simulink model "spe_engine_throttle1"  (R2020a)
settings: Solver=ode45  StartTime=0  StopTime=0.5  FixedStep=.001  RelTol=1e-3  EnableMultiTasking=on
PreLoadFcn:
  | load spe_engine_throttle1.mat
model workspace (MAT data in the model file):
  spe_engine_throttle1_spesession : sldodialogs.data.SessionData (value not decoded)
undefined symbols (not defined in the file): angle_init, angle_open, c, input_delay, J, k, Kt
settings Model: Creator=The MathWorks, Inc.  LastModifiedBy=GreHiDel
settings SolverCC: ZeroCrossAlgorithm=Classic  InsertRTBMode=Auto
settings DataIOCC: ExternalInput=[time1,input1]  LoadExternalInput=on  SaveFormat=Array  SaveOutput=off  SaveTime=off  ReturnWorkspaceOutputs=off
settings OptimizationCC: BooleanDataType=off  ExpressionDepthLimit=2147483647  InitFltsAndDblsToZero=on  LifeSpan=inf  BufferReusableBoundary=off
settings DebuggingCC: SaveWithParameterizedLinksMsg=none  UnderspecifiedInitializationDetection=Classic  MergeDetectMultiDrivingBlocksExec=none  SignalResolutionControl=TryResolveAllWithWarning  MultiTaskDSMMsg=warning  MultiTaskCondExecSysMsg=none  FcnCallInpInsideContextMsg=warning  BusObjectLabelMismatch=none  StateNameClashWarn=warning  SFUnexpectedBacktrackingDiag=warning  SFNoUnconditionalDefaultTransitionDiag=warning  SFExecutionAtInitializationDiag=none  ArithmeticOperatorsInVariantConditions=warning
settings HardwareCC: ProdBitPerPointer=32  ProdBitPerSizeT=32  ProdBitPerPtrDiffT=32  ProdLargestAtomicFloat=None  ProdIntDivRoundTo=Undefined  ProdEndianess=Unspecified  ProdWordSize=32  ProdHWDeviceType=32-bit Generic  TargetUnknown=on
settings ModelReferenceCC: PropagateSignalLabelsOutOfModel=off
settings CodeAppCC: StateflowObjectComments=on
settings GRTTargetCC: TargetFcnLib=ansi_tfl_tmw.mat  TargetLangStandard=C89/C90 (ANSI)  CombineOutputUpdateFcns=off  GRTInterface=on
settings ConfigComp: CovMetricSettings=dw  CovHtmlReporting=on  CovSaveCumulativeToWorkspaceVar=on  CovSaveSingleToWorkspaceVar=on

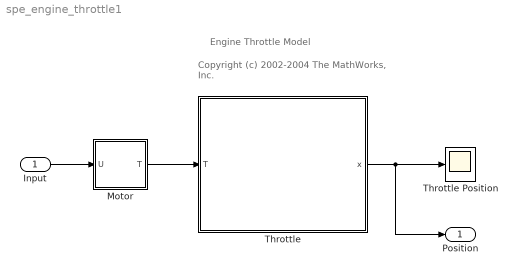
== system spe_engine_throttle1 ==
  note: Engine Throttle Model
  note: Copyright (c) 2002-2004 The MathWorks, Inc.
  Input : Inport
  Motor : Subsystem
  Throttle : Subsystem  mask{J=J, c=c, k=k, init=angle_init, open_val=angle_open}
      mask prompts: J "Inertia:"; c "Damping:"; k "Stiffness:"; init "Resting Angle:"; open_val "Open Angle:"
      mask init:
      | throttle = imread('spe_engine_throttle.jpg');
      mask Display: image(throttle)
  Throttle Position : Scope
  Position : Outport
  wires:
  Motor/1(T) -> Throttle/1(T)
  Input/1 -> Motor/1(U)
  Throttle/1(x) -> Throttle Position/1, Position/1

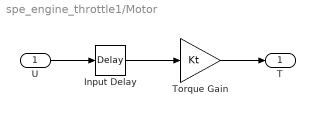
== system spe_engine_throttle1/Motor ==
  U : Inport
  Input Delay : TransportDelay  DelayTime=input_delay
  Torque Gain : Gain  Gain=Kt  SaturateOnIntegerOverflow=on  OutDataTypeStr=Inherit: Same as input  ParamDataTypeStr=Inherit: Same as input
  T : Outport
  wires:
  Input Delay/1 -> Torque Gain/1
  Torque Gain/1 -> T/1
  U/1 -> Input Delay/1

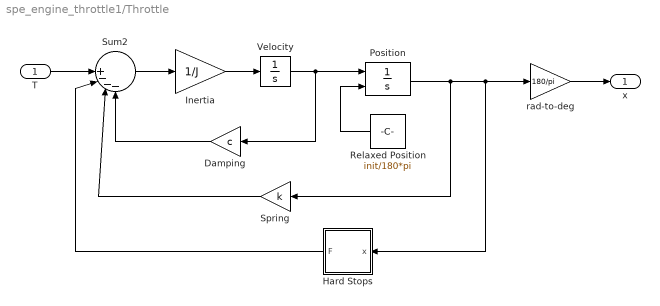
== system spe_engine_throttle1/Throttle ==
  T : Inport
  Damping : Gain  Gain=c
  Hard Stops : Subsystem  mask{H=open_val/180*pi, K=2.86e5, L=init/180*pi}
      mask prompts: H "Upper Limit:"; K "Stiffness:"; L "Lower Limit:"
  Inertia : Gain  Gain=1/J  SaturateOnIntegerOverflow=on  OutDataTypeStr=Inherit: Same as input  ParamDataTypeStr=Inherit: Same as input
  Position : Integrator  InitialConditionSource=external
  Relaxed Position : Constant  Value=init/180*pi
  Spring : Gain  Gain=k
  Sum2 : Sum  Inputs=|||+---  InputSameDT=on  SaturateOnIntegerOverflow=on  OutDataTypeStr=Inherit: Same as first input
  Velocity : Integrator
  rad-to-deg : Gain  Gain=180/pi
  x : Outport
  wires:
  Spring/1 -> Sum2/3
  Damping/1 -> Sum2/4
  Position/1 -> Hard Stops/1(x), rad-to-deg/1, Spring/1
  Sum2/1 -> Inertia/1
  Inertia/1 -> Velocity/1
  Velocity/1 -> Position/1, Damping/1
  T/1 -> Sum2/1
  rad-to-deg/1 -> x/1
  Relaxed Position/1 -> Position/2
  Hard Stops/1(F) -> Sum2/2

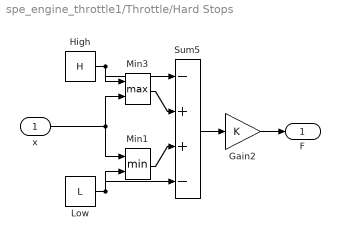
== system spe_engine_throttle1/Throttle/Hard Stops ==
  x : Inport
  Gain2 : Gain  Gain=K  SaturateOnIntegerOverflow=on  OutDataTypeStr=Inherit: Same as input  ParamDataTypeStr=Inherit: Same as input
  High : Constant  Value=H
  Low : Constant  Value=L
  Min1 : MinMax  Inputs=2  InputSameDT=on  SaturateOnIntegerOverflow=on
  Min3 : MinMax  Function=max  Inputs=2  InputSameDT=on  SaturateOnIntegerOverflow=on
  Sum5 : Sum  Inputs=-+||+-  InputSameDT=on  SaturateOnIntegerOverflow=on  OutDataTypeStr=Inherit: Same as first input
  F : Outport
  wires:
  Min1/1 -> Sum5/3
  Min3/1 -> Sum5/2
  High/1 -> Min3/1, Sum5/1
  Low/1 -> Sum5/4, Min1/2
  Sum5/1 -> Gain2/1
  x/1 -> Min3/2, Min1/1
  Gain2/1 -> F/1
